simulink model "rcm112_app"  (R2024a)
settings: Solver=FixedStepDiscrete  StartTime=0.0  StopTime=10.0  FixedStep=0.005  RelTol=1e-3  EnableMultiTasking=on
PreLoadFcn:
  | try, model_open; catch, disp('Error occurred while executing model pre-load callback: model_open.m'); disp('Please assure that the MATLAB working directory is set to the model directory before opening.'); end
InitFcn:
  | try, model_open; catch, end
undefined symbols (not defined in the file or in its folder): dataName, enumName, enumValue, raptor_get_safe_string, raptor_xcp_function, RCM
libraries: Raptor_lib x57, simulink x14, simulink_extras x4
(part 1 of 2)
CloseFcn:
  | try, model_close; catch, end
settings Model: Raptor_Target=RCM-58NN-112-2202  Raptor_Calloc=NonVolatile (EEPROM)  RaptorUIDSize=4  RaptorBuildNum=1  Raptor_ecuaddr=11  Creator=mstewart  LastModifiedBy=mstewart
settings SolverCC: AlgebraicLoopSolver=TrustRegion
settings DataIOCC: LimitDataPoints=on  SaveFormat=Array  SignalLoggingSaveFormat=ModelDataLogs  ReturnWorkspaceOutputs=off
settings OptimizationCC: DefaultParameterBehavior=Inlined  ExpressionDepthLimit=2147483647  InitFltsAndDblsToZero=on  LifeSpan=1  EfficientTunableParamExpr=on
settings DebuggingCC: SolverPrmCheckMsg=warning  InheritedTsInSrcMsg=none  FcnCallInpInsideContextMsg=warning  UnconnectedInputMsg=warning  UnconnectedOutputMsg=warning  UnconnectedLineMsg=warning  StateNameClashWarn=warning  SFUnexpectedBacktrackingDiag=warning  SFNoUnconditionalDefaultTransitionDiag=warning  SFExecutionAtInitializationDiag=none  ArithmeticOperatorsInVariantConditions=warning
settings HardwareCC: ProdBitPerPointer=32  ProdBitPerSizeT=32  ProdBitPerPtrDiffT=32  ProdLargestAtomicInteger=Long  ProdLargestAtomicFloat=Double  ProdEndianess=BigEndian  ProdWordSize=32  ProdHWDeviceType=Freescale->MPC55xx  TargetIntDivRoundTo=Zero  TargetEndianess=BigEndian  ProdEqTarget=off
settings ModelReferenceCC: EnableRefExpFcnMdlSchedulingChecks=on  PropagateSignalLabelsOutOfModel=off
settings SFSimCC: SimUseLocalCustomCode=off  MATLABDynamicMemAlloc=off  CustomCodeUndefinedFunction=UseInterfaceOnly
settings RTWCC: Description=Raptor (tm)  SystemTargetFile=raptor.tlc  GenCodeOnly=on  MakeCommand=raptor_make_rtw  TemplateMakefile=raptor.tmf  RTWUseLocalCustomCode=off  GPUComputeCapability=3.5  DLArmComputeVersion=19.05
settings CodeAppCC: IgnoreCustomStorageClasses=off  MaxIdLength=100  CustomSymbolStrType=$N$R$M  StateflowObjectComments=on  InternalIdentifier=Classic
settings STFCustomTargetCC: TargetLangStandard=C89/C90 (ANSI)  CodeReplacementLibrary=No Double Hardware Support  GenerateSampleERTMain=on  ModelReferenceCompliant=off  CombineOutputUpdateFcns=on  ERTCustomFileBanners=on  SupportContinuousTime=off  SupportNonInlinedSFcns=off  RemoveResetFunc=on  MATLABClassNameForMDSCustomization=Simulink.SoftwareTarget.ERTCustomization  GRTInterface=off  UseToolchainInfoCompliant=off  SystemTargetFile=raptor.tlc
settings ERTTargetCC: CodeReplacementLibrary=No Double Hardware Support  MultiwordLength=2048  GenerateSampleERTMain=on  ModelReferenceCompliant=off  ParMdlRefBuildCompliant=off  CompOptLevelCompliant=off  ConcurrentExecutionCompliant=off  ModelStepFunctionPrototypeControlCompliant=off  CPPClassGenCompliant=off  UseToolchainInfoCompliant=off  ExtModeMexFile=noextcomm  InlinedParameterPlacement=NonHierarchical  ERTCustomFileTemplate=example_file_process.tlc  ConvertIfToSwitch=off  SuppressUnreachableDefaultCases=off
settings ConfigComp: CovMetricSettings=dw  CovSaveCumulativeToWorkspaceVar=on  CovSaveSingleToWorkspaceVar=on  CovExternalEMLEnable=off  CovSFcnEnable=off

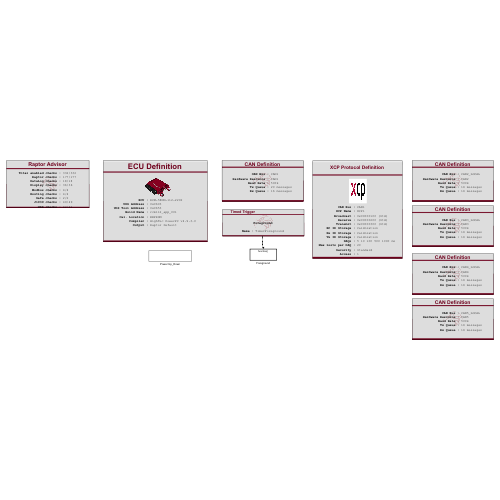
[thumbnail: Simulink's stored preview of the top-level diagram]
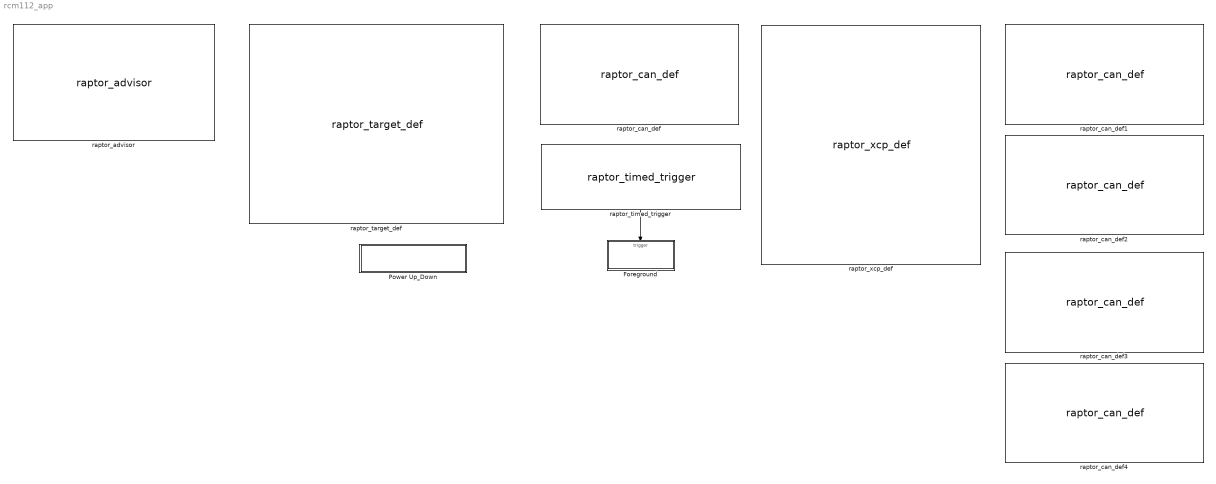
== system rcm112_app ==
  Foreground : Subsystem  TreatAsAtomicUnit=on
      settings: RTWSystemCode=Nonreusable function
  Power Up_Down : Subsystem  mask{group='Diagnostics | Power Up_Down'}
  raptor_advisor : Raptor_lib/Configuration/raptor_advisor  pop_setEnable=Enable All  ckb_Raptor=on  ckb_AppMonitor=on  tbl_AppMonitor={ 'on', 'App Monitor'; 'on', 'App Monitor Measurement'; 'on', 'App Monitor Stop'; 'on', 'Reboot'; 'on', 'Task Monitor'; 'on', 'Task Monitor Measurement' }  ckb_CAN=on  tbl_CAN={ 'on', 'CAN Baud Rate'; 'on', 'CAN Bus Off Recovery'; 'on', 'CAN Definition'; 'on', 'CAN Hardware Mailbox Config'; 'on', 'CAN Mailbox Properties'; 'on', 'CAN Partial Networking'; 'on', 'CAN Queue Info'; 'on', 'CAN Rx Message'; 'on', 'CAN Rx Raw'; 'on', 'CAN State'; 'on', 'CAN Trigger'; 'on', 'CAN Tx Message'; 'on', 'CAN Tx Raw'; 'on', 'CAN/FD Definition'; 'on', 'CAN/FD Rx Message'; 'on', 'CAN/FD Rx Raw'; 'on', 'CAN/FD Tx Message'; 'on', 'CAN/FD Tx Raw'; 'on', 'Custom Baud Rate'; 'on', 'DBC Pack'; 'on', 'DBC Unpack' }  ckb_Checksum=on  tbl_Checksum={ 'on', 'Calculate Checksum'; 'on', 'Read Checksum' }  ckb_Config=on  tbl_Config={ 'on', 'Configuration Read'; 'on', 'System Variable Access Level'; 'on', 'ECU Definition'; 'on', 'Set Target Address'; 'on', 'XCP Custom Security Seed/Key'; 'on', 'XCP Custom Security Trigger'; 'on', 'XCP Protocol Definition'; 'on', 'XCP Query'; 'on', 'XCP Set Address' }  ckb_DataStore=on  tbl_DataStore={ 'on', 'Adjustment'; 'on', 'Data Store'; 'on', 'Data Read'; 'on', 'Data Write'; 'on', 'Load NonVolatile Defaults'; 'on', 'Fixed NV Manager'; 'on', 'Measurement'; 'on', 'Memory Read'; 'on', 'NonVolatile Settings'; 'on', 'Override'; 'on', 'Fixed NonVolatile Status'; 'on', 'NonVolatile Status'; 'on', 'Store NonVolatile' }  ckb_Engine=on  tbl_Engine={ 'on', 'Angle Time'; 'on', 'CamShaft Sensor Info'; 'on', 'Encoder Def'; 'on', 'Injector Output'; 'on', 'Knock Results'; 'on', 'Knock Input'; 'on', 'Spark Output'; 'on', 'Wideband O2 Input' }  ckb_Ethernet=on  tbl_Ethernet={ 'on', 'Ethernet Adapter Get MAC Address'; 'on', 'Ethernet Definition'; 'on', 'Ethernet Interface Definition'; 'on', 'Ethernet Interface Get VLAN'; 'on', 'Ethernet Interface Set VLAN'; 'on', 'Ethernet Socket - TCP Server'; 'on', 'Ethernet Socket - UDP Server'; 'on', 'Ethernet Socket State'; 'on', 'Ethernet TCP Accept'; 'on', 'Ethernet TCP Close'; 'on', 'Ethernet TCP Connect'; 'on', 'Ethernet TCP Listen'; 'on', 'Ethernet TCP Receive'; 'on', 'Ethernet TCP Send'; 'on', 'Ethernet TCP Shutdown'; 'on', 'Ethernet UDP Multicast Join'; 'on', 'Ethernet UDP Multicast Leave'; 'on', 'Ethernet UDP Receive'; 'on', 'Ethernet UDP Send' }  ckb_OBD_Faults=on  tbl_OBD_Faults={ 'on', 'OBD Counter'; 'on', 'Increment OBD Counter'; 'on', 'Read OBD Counter'; 'on', 'Reset OBD Counter'; 'on', 'Drive Cycle Complete'; 'on', 'OBD Ratio'; 'on', 'Increment OBD Ratio'; 'on', 'Read OBD Ratio'; 'on', 'Reset OBD Ratio' }  ckb_Faults=on  tbl_Faults={ 'on', 'Fault Action'; 'on', 'Fault Action Iterator'; 'on', 'Fault Action Read'; 'on', 'Clear Fault'; 'on', 'Fault Data'; 'on', 'Fault Data Read'; 'on', 'Fault Data Write'; 'on', 'Fault'; 'on', 'Fault Handle'; 'on', 'Fault Iterator'; 'on', 'Fault Manager'; 'on', 'Fault Measurement'; 'on', 'Null Fault'; 'on', 'Fault Config'; 'on', 'Fault Reference'; 'on', 'Set Fault State'; 'on', 'Fault State Iterator'; 'on', 'Fault Status'; 'on', 'Fault Trigger'; 'on', 'Fault State Count' }  ckb_IO=on  tbl_IO={ 'on', 'Analog Input'; 'on', 'Analog Input Reference'; 'on', 'Analog Output'; 'on', 'Device Diagnostics'; 'on', 'Digital Input'; 'on', 'Digital Output'; 'on', 'Frequency Input'; 'on', 'H-Bridge Output'; 'on', 'IMU Calibrate'; 'on', 'IMU Reset'; 'on', 'IMU Status'; 'on', 'Inertial Measurement'; 'on', 'Input Capture Defn'; 'on', 'Input Capture Get'; 'on', 'Input Capture Trigger'; 'on', 'Input Status'; 'on', 'Internal Measurement'; 'on', 'Output Status'; 'on', 'PWM Output'; 'on', 'Quadrature Input'; 'on', 'Set Hardware Option'; 'on', 'Set Input Option'; 'on', 'Temperature Measurement' }  ckb_LIN=on  tbl_LIN={ 'on', 'LIN Master Definition'; 'on', 'LIN Get Schedule'; 'on', 'LIN Rx Message'; 'on', 'LIN Set Schedule'; 'on', 'LIN Slave Definition'; 'on', 'LIN State'; 'on', 'LIN Trigger'; 'on', 'LIN Tx Message' }  ckb_SENT=on  tbl_SENT={ 'on', 'SENT Definition'; 'on', 'SENT Receive State' }  ckb_Serial=on  tbl_Serial={ 'on', 'Serial Definition'; 'on', 'Serial Rx'; 'on', 'Serial Trigger'; 'on', 'Serial Tx' }  ckb_Strings=on  tbl_Strings={ 'on', 'String'; 'on', 'Arr 2 Str'; 'on', 'String Length'; 'on', 'Printf'; 'on', 'String Reference'; 'on', 'scanf'; 'on', 'Str 2 Arr' }  ckb_Tables=on  tbl_Tables={ 'on', 'Table Adapt'; 'on', 'Axis'; 'on', 'Axis Reference'; 'on', 'Table Interpolate 1D'; 'on', 'Table Interpolate 1D Reference'; 'on', 'Table Interpolate 2D'; 'on', 'Table Interpolate 2D Reference' }  ckb_Time=on  tbl_Time={ 'on', 'Datetime Conversion In'; 'on', 'Datetime Conversion Out'; 'on', 'Real Time Clock Read'; 'on', 'Real Time Clock Set' }  ckb_Triggers=on  tbl_Triggers={ 'on', 'App Trigger'; 'on', 'dT'; 'on', 'Distributed Action Defn'; 'on', 'Distributed Action Execute'; 'on', 'Distributed Action Trigger'; 'on', 'Shutdown'; 'on', 'Sleep'; 'on', 'Startup'; 'on', 'Time'; 'on', 'Timed Trigger'; 'on', 'Timed Trigger Config'; 'on', 'Define Trigger'; 'on', 'Trigger Execute'; 'on', 'Output Trigger Reference'; 'on', 'Trigger Select' }  ckb_DataLog=on  tbl_DataLog={ 'on', 'Data Log Erase'; 'on', 'Data Log Read'; 'on', 'Data Log Write'; 'on', 'File Close'; 'on', 'File EOF'; 'on', 'File Exists'; 'on', 'File Get Free Space'; 'on', 'File Open'; 'on', 'File Position'; 'on', 'File Read'; 'on', 'File Remove'; 'on', 'File Rename'; 'on', 'File Seek'; 'on', 'File Size'; 'on', 'File Sync'; 'on', 'USB Eject'; 'on', 'USB Status'; 'on', 'File Write' }  ckb_Display=on  ckb_Drawing=on  tbl_Drawing={ 'on', 'Clear Rect'; 'on', 'Clear Screen'; 'on', 'Draw Arc'; 'on', 'Draw Button'; 'on', 'Draw Circle'; 'on', 'Draw Image'; 'on', 'Draw Line'; 'on', 'Draw Polygon'; 'on', 'Draw Rectangle'; 'on', 'Draw Text'; 'on', 'Element'; 'on', 'Fill Circle'; 'on', 'Fill Ellipse'; 'on', 'Fill Polygon'; 'on', 'Fill Rect'; 'on', 'Image Ref' }  ckb_Menu=on  tbl_Menu={ 'on', 'Menu Screen Definition'; 'on', 'Menu Sel Item'; 'on', 'Menu Text'; 'on', 'Menu Title' }  ckb_Prefab=on  tbl_Prefab={ 'on', 'Gauge: Create'; 'on', 'Gauge: Update' }  ckb_ScreenFuncs=on  tbl_ScreenFuncs={ 'on', 'Hide Buttonbar'; 'on', 'Button Bar Properties'; 'on', 'Setup Button'; 'on', 'Goto Screen'; 'on', 'Recalibrate Screen'; 'on', 'Screen Definition'; 'on', 'Screen Reference'; 'on', 'Screen Select'; 'on', 'Splash Screen' }  ckb_Touchscreen=on  tbl_Touchscreen={ 'on', 'Button Status'; 'on', 'Display Touchscreen'; 'on', 'Button Def'; 'on', 'Hot Area Actions'; 'on', 'Update Swipe Action' }  ckb_Modbus=on  tbl_Modbus={ 'on', 'Modbus Master'; 'on', 'Modbus Slave'; 'on', 'Modbus Slave Error'; 'on', 'Modbus Slave Response' }  ckb_Routing=on  tbl_Routing={ 'on', 'J1939 Message Router'; 'on', 'Message Hardware Filter'; 'on', 'Message Network'; 'on', 'Message Router' }  ckb_Safe=on  tbl_Safe={ 'on', 'Raptor Stack Check'; 'on', 'Raptor Time Check' }  ckb_J1939=on  ckb_DMA=on  tbl_DMA={ 'on', 'DM14/15/16 Definition: DM14 Rx'; 'on', 'DM14/15/16 Definition: DM15 Rx'; 'on', 'DM14/15/16 Definition: DM15 Tx'; 'on', 'DM14/15/16 Definition: DMA Manager'; 'on', 'DMA Address Space Definition'; 'on', 'DMA Address Space Return'; 'on', 'DMA Address Space Trigger'; 'on', 'DMA Key'; 'on', 'DMA Key Trigger' }  ckb_DM_Msgs=on  tbl_DM_Msgs={ 'on', 'DM4 Transmit'; 'on', 'DM5 Transmit'; 'on', 'DM8 Transmit'; 'on', 'DM19 Transmit'; 'on', 'DM20 Transmit'; 'on', 'DM21 Transmit'; 'on', 'DM22 Rx Trigger'; 'on', 'DM24 Transmit'; 'on', 'DM25 Transmit'; 'on', 'DM26 Transmit'; 'on', 'DM29 Transmit'; 'on', 'DM30 Transmit'; 'on', 'DM33 Transmit'; 'on', 'DM34 Transmit'; 'on', 'DTC Transmit' }  ckb_EFF=on  tbl_EFF={ 'on', 'Clear Expanded FF'; 'on', 'Write Expanded FF'; 'on', 'Expanded FF Status' }  ckb_PGN_Tx=on  tbl_PGN_Tx={ 'on', 'CBI Transmit'; 'on', 'CI Transmit'; 'on', 'EC1 Transmit'; 'on', 'ECUID Transmit'; 'on', 'GTFI Transmit'; 'on', 'LTFI Transmit'; 'on', 'RC Transmit'; 'on', 'SOFT Transmit'; 'on', 'TTI2 Transmit'; 'on', 'VI Transmit' }  ckb_SPN=on  tbl_SPN={ 'on', 'SPN Read'; 'on', 'SPN Write' }  ckb_J1939_TP=on  tbl_J1939_TP={ 'on', 'J1939 DTC Rx Handler'; 'on', 'Source Addr'; 'on', 'PGN Enable'; 'on', 'PGN Request Slot'; 'on', 'PGN Enable'; 'on', 'PGN Trigger'; 'on', 'Tx ACK/NACK'; 'on', 'J1939 Protocol'; 'on', 'J1939 Transport Protocol Receive'; 'on', 'PGN Rx Trigger' }  ckb_UDS=on  ckb_ISO14229=on  tbl_ISO14229={ 'on', 'ISO14229 Custom Service 0x31'; 'on', 'ISO14229 Service 0x10 - Session Control'; 'on', 'ISO14229 Service 0x11 - ECU Reset'; 'on', 'ISO14229 Service 0x14 - Clear Diagnostic Information'; 'on', 'ISO14229 Service 0x19 - Read DTC Information'; 'on', 'ISO14229 Service 0x19 - Extended Data Definition'; 'on', 'ISO14229 Service 0x19 - Snapshot Record Definition'; 'on', 'ISO14229 Service 0x19 - Snapshot Record Clear'; 'on', 'ISO14229 Service 0x19 - Snapshot Record Clear All'; 'on', 'ISO14229 Service 0x19 - Snapshot Record Get'; 'on', 'ISO14229 Service 0x19 - Snapshot Record Set'; 'on', 'ISO14229 Service 0x22 - Read Data by Identifier'; 'on', 'ISO14229 Service 0x27 - Security Access'; 'on', 'ISO14229 Service 0x28 - Communication Control'; 'on', 'ISO14229 Service 0x2E - Write Data by Identifier'; 'on', 'ISO14229 Service 0x2F - Input Output by Identifier'; 'on', 'ISO14229 Service 0x2F - Input Output by Identifier Reset State'; 'on', 'ISO14229 Service 0x31 - Routine Control by Identifier'; 'on', 'ISO14229 Service 0x85 - DTC Control Setting' }  ckb_ISO15031=on  tbl_ISO15031={ 'on', 'ISO15031 Custom Service'; 'on', 'ISO15031 Service 0x01'; 'on', 'ISO15031 Service 0x03 - Emission-related diagnostic trouble codes'; 'on', 'ISO15031 Service 0x04 - Clear Diagnostic Information'; 'on', 'ISO15031 Service 0x07 - Emission-related pending diagnostic trouble codes'; 'on', 'ISO15031 Service 0x09 - Calibration Identification'; 'on', 'ISO15031 Service 0x09 - Calibration Verification Numbers'; 'on', 'ISO15031 Service 0x09 - ECU Name'; 'on', 'ISO15031 Service 0x09 - Request Vehicle Information'; 'on', 'ISO15031 Service 0x09 - Vehicle Identification Number'; 'on', 'ISO15031 Service 0x0A - Emission-related diagnostic trouble codes with permanent status' }  ckb_ISO15765=on  tbl_ISO15765={ 'on', 'ISO15765 Protocol Receive Queue Info'; 'on', 'ISO15765 Protocol Transmit Queue Info'; 'on', 'ISO15765 Protocol Transmit Raw' }  ckb_UDS_Basics=on  tbl_UDS_Basics={ 'on', 'UDS Client Functional Address Request'; 'on', 'UDS Client Functional Address Request Send'; 'on', 'UDS Protocol Client Request Raw'; 'on', 'UDS Protocol Receive Raw'; 'on', 'UDS Protocol Transmit Raw'; 'on', 'UDS Server Service Process Raw' }  ckb_UDS_Other=on  tbl_UDS_Other={ 'on', 'ISO13400 DoIP Entity'; 'on', 'UDS Protocol'; 'on', 'UDS Set Buffer Storage' }
      settings: SourceProductName=Raptor
  raptor_can_def : Raptor_lib/CAN/raptor_can_def  canBus='CAN1'  resourceValues=CAN5|CAN1|CAN2|CAN3|CAN4|(None)  resource=CAN1  baudRateValues=33k|50k|100k|125k|200k|250k|333k|500k|667k|800k|1000k|500k_80%SP|500k_81%SP  baudRate=500k  enable_baud_rate_config=0  sim_func_name='ConfigureCANBaudRate'  createButton=0  txQueueSize=20  rxQueueSize=16  useCustomBR=0  customBR='CustomBaudRate'  updateButton=0
      settings: SourceProductName=Raptor
  raptor_can_def1 : Raptor_lib/CAN/raptor_can_def  canBus='CAN2_LOCAL'  resourceValues=CAN5|CAN1|CAN2|CAN3|CAN4|(None)  resource=CAN2  baudRateValues=33k|50k|100k|125k|200k|250k|333k|500k|667k|800k|1000k  baudRate=500k  enable_baud_rate_config=0  sim_func_name='ConfigureCANBaudRate'  createButton=[]  txQueueSize=16  rxQueueSize=16  useCustomBR=0  customBR='CustomBaudRate'  updateButton=[]
      settings: SourceProductName=Raptor
  raptor_can_def2 : Raptor_lib/CAN/raptor_can_def  canBus='CAN3_LOCAL'  resourceValues=CAN5|CAN1|CAN2|CAN3|CAN4|(None)  resource=CAN3  baudRateValues=33k|50k|100k|125k|200k|250k|333k|500k|667k|800k|1000k  baudRate=500k  enable_baud_rate_config=0  sim_func_name='ConfigureCANBaudRate'  createButton=[]  txQueueSize=16  rxQueueSize=16  useCustomBR=0  customBR='CustomBaudRate'  updateButton=[]
      settings: SourceProductName=Raptor
  raptor_can_def3 : Raptor_lib/CAN/raptor_can_def  canBus='CAN4_LOCAL'  resourceValues=CAN5|CAN1|CAN2|CAN3|CAN4|(None)  resource=CAN4  baudRateValues=33k|50k|100k|125k|200k|250k|333k|500k|667k|800k|1000k  baudRate=500k  enable_baud_rate_config=0  sim_func_name='ConfigureCANBaudRate'  createButton=[]  txQueueSize=16  rxQueueSize=16  useCustomBR=0  customBR='CustomBaudRate'  updateButton=[]
      settings: SourceProductName=Raptor
  raptor_can_def4 : Raptor_lib/CAN/raptor_can_def  canBus='CAN5_LOCAL'  resourceValues=CAN5|CAN1|CAN2|CAN3|CAN4|(None)  resource=CAN5  baudRateValues=33k|50k|100k|125k|200k|250k|333k|500k|667k|800k|1000k  baudRate=500k  enable_baud_rate_config=0  sim_func_name='ConfigureCANBaudRate'  createButton=[]  txQueueSize=16  rxQueueSize=16  useCustomBR=0  customBR='CustomBaudRate'  updateButton=[]
      settings: SourceProductName=Raptor
  raptor_target_def : Raptor_lib/Configuration/raptor_target_def  targetValues=BCM-5606B-060-2201|BCM-5646-48-1404|CSM-S32K148-030-1903|DISP-VC128-1901|DISP-VC320L-1402|DISP-VC320-1204|DISP-VC800-1402|DISP-VC500-1904|DISP-VC700-2003|DISP-VC300R-2004|GCM-5634M-070-1459|GCM-5634M-070-1559|GCM-5634M-070-1562|ECM-1793-196-1503|GCM-1793-196-1503|GCM-5605B-048-1906|GCM-5605B-048-2104|GCM-5607B-80-1901|GCM-5607B-80-1903|GCM-5607B-80-2001|RCM-5743R-080-2005|RCM-5743R-080-2106|RCM-5743R-080-2203|UAS-5743R-047-2102|UAS-5743R-047-2107|GCM-5746R-048-1902|RCM-58NN-112-2007|RCM-58NN-112-2103|RCM-58NN-112-2202|HCM-5604-36-1303|HCM-5604-36-1702  target=RCM-58NN-112-2202  simpack=0  simulator=0  heap=4*1024  stack=2*1024  fgndStack=3*1024  bgndStack=2*1024  idleStack=1024  intStack=1536  sdStack=1024  appStack=1024  ecuaddr=11  uds_server_addr_ext=0  uds_server_addr=hex2dec('603')  uds_client_addr=hex2dec('653')  callocValues=Constant (FLASH)|NonVolatile (EEPROM)  calloc=NonVolatile (EEPROM)  compilerValues=HighTec PowerPC v4.9.3.0|SPC5Studio-6.0.0-Green  compiler=HighTec PowerPC v4.9.3.0  setFileName=0  exeName=[raptor_get_safe_string(bdroot) '_']  addBuildNum=1  minVerChars=3  extraOutput=0  buildLocationValues=Raptor Default|Model Directory|User Defined  buildLocation=Raptor Default  exeLocation=''  exeFileButton=0  a2lLocation=''  a2lFileButton=0  rpgLocation=''  rpgFileButton=0
      settings: SourceProductName=Raptor
  raptor_timed_trigger : Raptor_lib/Triggers/raptor_timed_trigger  triggerValues=Task_Core0_1ms|Task_Core0_5ms|Task_Core0_10ms|Task_Core0_20ms|Task_Core0_50ms|Task_Core0_100ms|Task_Core0_250ms|Task_Core0_500ms|Second|Minute|Foreground|Background  trigger=Foreground  inherited=0  alwaysEnabled=1  triggerPriority=0  triggerName=Foreground
      settings: SourceProductName=Raptor
  raptor_xcp_def : Raptor_lib/Configuration/raptor_xcp_def  XCPname='XCP1'  canBus='CAN1'  bcID=hex2dec('100')  bcID_TypeValues=Standard|Extended  bcID_Type=Standard  rxID=hex2dec('200')  rxID_TypeValues=Standard|Extended  rxID_Type=Standard  txID=hex2dec('300')  txID_TypeValues=Standard|Extended  txID_Type=Standard  daqRates=[5 10 100 500 1000]  numODTs=20  genCANAPE=0  genVISION=0  securityValues=Standard|None|Custom User Defined|LoopEnergy  security=Standard  dllName=raptor_XCPSecurity.dll  accessValues=4|3|2|1  access=1  bcStorageValues=Constant (FLASH)|NonVolatile (EEPROM)|FixedNonVolatile (EEPROM)|Volatile (RAM)|Calibration  bcStorage=Calibration  txStorageValues=Constant (FLASH)|NonVolatile (EEPROM)|FixedNonVolatile (EEPROM)|Volatile (RAM)|Calibration  txStorage=Calibration  rxStorageValues=Constant (FLASH)|NonVolatile (EEPROM)|FixedNonVolatile (EEPROM)|Volatile (RAM)|Calibration  rxStorage=Calibration
      settings: SourceProductName=Raptor
  wires:
  raptor_timed_trigger/1 -> Foreground/Trigger

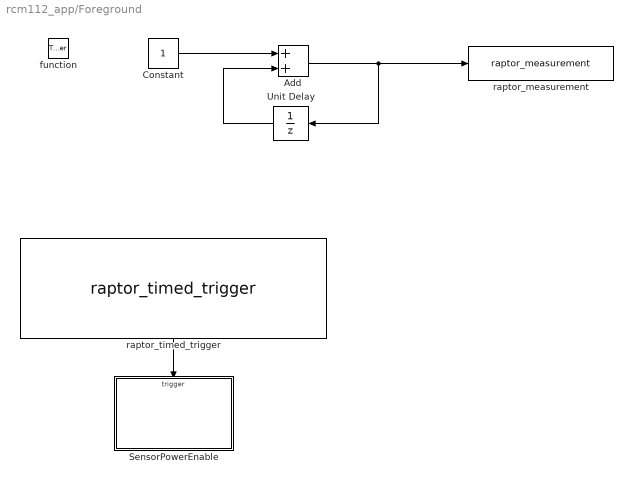
== system rcm112_app/Foreground ==
  function : TriggerPort  TriggerType=function-call  VariantControl=Variant
  Add : Sum
  Constant : Constant
  SensorPowerEnable : Subsystem
  Unit Delay : UnitDelay  SampleTime=-1  HasFrameUpgradeWarning=on
  raptor_measurement : Raptor_lib/Data Storage/raptor_measurement  paramName='Counter'  nameSource=Parameter  calDispType=Number  calEnum={'False', 'True'}  calGain=1.0  calOffset=0.0  calMax=inf  calMin=-inf  calFormat='-1'  calUnit=''  calHelp=''  calAccess=4  calFunction=raptor_xcp_function(gcb)  calVisible=on
      settings: SourceProductName=Raptor
  raptor_timed_trigger : Raptor_lib/Triggers/raptor_timed_trigger  triggerValues=Task_Core0_1ms|Task_Core0_Fgnd|Task_Core0_20ms|Task_Core0_50ms|Task_Core0_100ms|Task_Core0_250ms|Task_Core0_500ms|Second|Minute|Foreground|Foregroundx2|Foregroundx5|Foregroundx10|Foregroundx20|Background|Backgroundx2|Backgroundx5|Backgroundx10|Backgroundx20  trigger=Task_Core0_Fgnd  inherited=1  alwaysEnabled=1  triggerPriority=0  triggerName=FGND_10MS_SensPower
      settings: SourceProductName=Raptor
  wires:
  Constant/1 -> Add/1
  Add/1 -> raptor_measurement/1, Unit Delay/1
  Unit Delay/1 -> Add/2
  raptor_timed_trigger/1 -> SensorPowerEnable/Trigger

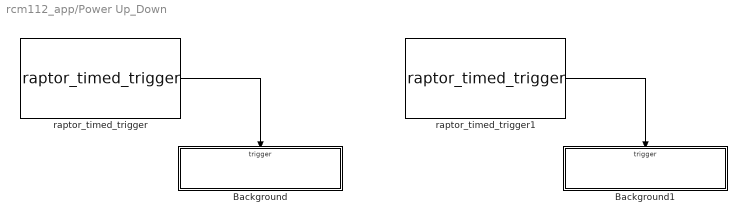
== system rcm112_app/Power Up_Down ==
  Background : Subsystem  mask{group='System | Power Up_Down', samptime=.05}
      mask prompts: samptime "Sample Time"
      mask Display: disp(['Sample Time:\n' num2str(samptime)])
  Background1 : Subsystem
  raptor_timed_trigger : Raptor_lib/Triggers/raptor_timed_trigger  triggerValues=Task_Core0_1ms|Task_Core0_5ms|Task_Core0_10ms|Task_Core0_20ms|Task_Core0_50ms|Task_Core0_100ms|Task_Core0_250ms|Task_Core0_500ms|Second|Minute|Foreground|Background  trigger=Background  inherited=0  alwaysEnabled=1  triggerPriority=50  triggerName=Background_50MS
      settings: SourceProductName=Raptor
  raptor_timed_trigger1 : Raptor_lib/Triggers/raptor_timed_trigger  triggerValues=Task_Core0_1ms|Task_Core0_5ms|Task_Core0_10ms|Task_Core0_20ms|Task_Core0_50ms|Task_Core0_100ms|Task_Core0_250ms|Task_Core0_500ms|Second|Minute|Foreground|Background  trigger=Background  inherited=0  alwaysEnabled=1  triggerPriority=51  triggerName=Background_50MS_SBN1H
      settings: SourceProductName=Raptor
  wires:
  raptor_timed_trigger/1 -> Background/Trigger
  raptor_timed_trigger1/1 -> Background1/Trigger

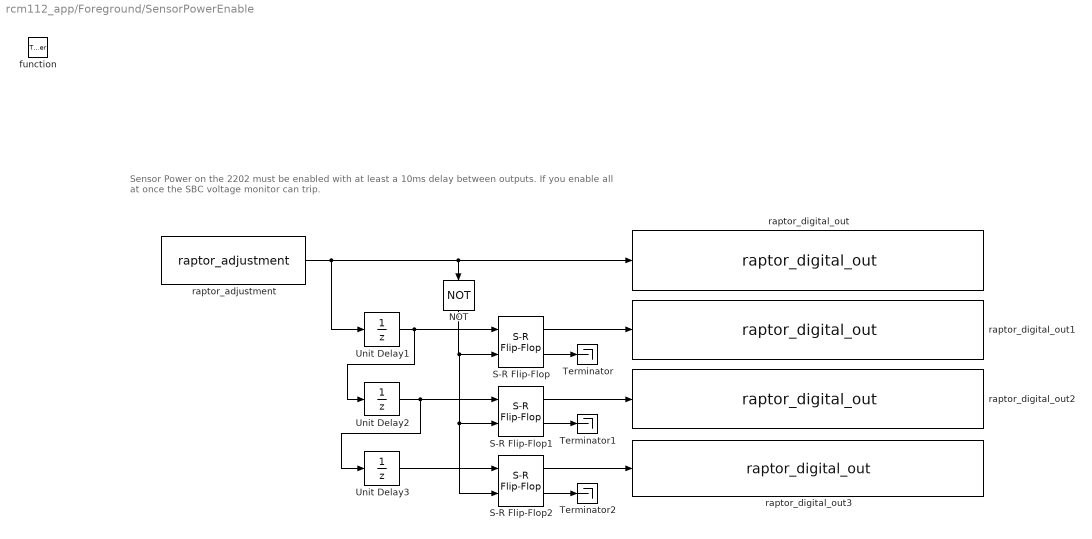
== system rcm112_app/Foreground/SensorPowerEnable ==
  note: Sensor Power on the 2202 must be enabled with at least a 10ms delay between outputs. If you enable all at once the SBC voltage monitor can trip.
  function : TriggerPort  TriggerType=function-call  VariantControl=Variant
  NOT : Logic  Operator=NOT
  S-R Flip-Flop : simulink_extras/Flip Flops/S-R Flip-Flop  initial_condition=0
  S-R Flip-Flop1 : simulink_extras/Flip Flops/S-R Flip-Flop  initial_condition=0
  S-R Flip-Flop2 : simulink_extras/Flip Flops/S-R Flip-Flop  initial_condition=0
  Terminator : Terminator
  Terminator1 : Terminator
  Terminator2 : Terminator
  Unit Delay1 : UnitDelay  SampleTime=-1  HasFrameUpgradeWarning=on
  Unit Delay2 : UnitDelay  SampleTime=-1  HasFrameUpgradeWarning=on
  Unit Delay3 : UnitDelay  SampleTime=-1  HasFrameUpgradeWarning=on
  raptor_adjustment : Raptor_lib/Data Storage/raptor_adjustment  paramName='SensorPowerEnable'  nameSource=Parameter  initValue=false  dataType=boolean  storage=Calibration  calDispType=Enumeration  calEnum={'False', 'True'}  calGain=1.0  calOffset=0.0  calMax=inf  calMin=-inf  calFormat='-1'  calUnit=''  calHelp=''  calAccess=1  calFunction='Enables'  calDispHeaders=off  calColHeaders={'Col1' 'Col2' 'Col3'}  calRowHeaders={'Row1' 'Row2' 'Row3'}
      settings: SourceProductName=Raptor
  raptor_digital_out : Raptor_lib/Input & Output/raptor_digital_out  resourceValues=SENSOR_POWER_A_EN|SENSOR_POWER_B_EN|SENSOR_POWER_C_EN|SENSOR_POWER_D_EN|LSO1|MPRD_EN|POWER_HOLD|(None)  resource=SENSOR_POWER_A_EN  driverTypeValues=Enable  driverType=Enable
      settings: SourceProductName=Raptor
  raptor_digital_out1 : Raptor_lib/Input & Output/raptor_digital_out  resourceValues=SENSOR_POWER_A_EN|SENSOR_POWER_B_EN|SENSOR_POWER_C_EN|SENSOR_POWER_D_EN|LSO1|MPRD_EN|POWER_HOLD|(None)  resource=SENSOR_POWER_B_EN  driverTypeValues=Enable  driverType=Enable
      settings: SourceProductName=Raptor
  raptor_digital_out2 : Raptor_lib/Input & Output/raptor_digital_out  resourceValues=SENSOR_POWER_A_EN|SENSOR_POWER_B_EN|SENSOR_POWER_C_EN|SENSOR_POWER_D_EN|LSO1|MPRD_EN|POWER_HOLD|(None)  resource=SENSOR_POWER_C_EN  driverTypeValues=Enable  driverType=Enable
      settings: SourceProductName=Raptor
  raptor_digital_out3 : Raptor_lib/Input & Output/raptor_digital_out  resourceValues=SENSOR_POWER_A_EN|SENSOR_POWER_B_EN|SENSOR_POWER_C_EN|SENSOR_POWER_D_EN|LSO1|MPRD_EN|POWER_HOLD|(None)  resource=SENSOR_POWER_D_EN  driverTypeValues=Enable  driverType=Enable
      settings: SourceProductName=Raptor
  wires:
  S-R Flip-Flop/1 -> raptor_digital_out1/1
  Unit Delay1/1 -> S-R Flip-Flop/1, Unit Delay2/1
  raptor_adjustment/1 -> NOT/1, raptor_digital_out/1, Unit Delay1/1
  NOT/1 -> S-R Flip-Flop2/2, S-R Flip-Flop1/2, S-R Flip-Flop/2
  S-R Flip-Flop/2 -> Terminator/1
  S-R Flip-Flop1/2 -> Terminator1/1
  S-R Flip-Flop2/1 -> raptor_digital_out3/1
  S-R Flip-Flop1/1 -> raptor_digital_out2/1
  Unit Delay2/1 -> S-R Flip-Flop1/1, Unit Delay3/1
  Unit Delay3/1 -> S-R Flip-Flop2/1
  S-R Flip-Flop2/2 -> Terminator2/1

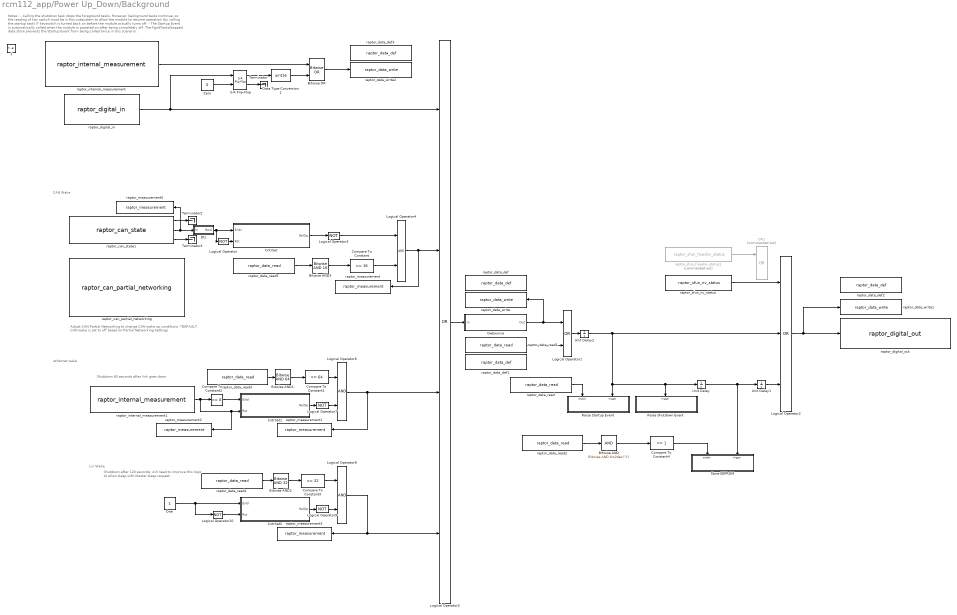
== system rcm112_app/Power Up_Down/Background ==
  note: Shutdown 60 seconds after link goes down
  note: ethernet wake
  note: Notes :
      | - Calling the shutdown task stops the foreground tasks. However, background tasks continue, so the reading of key switch must be in this subsystem to allow the module
      | to resume operation (by calling the startup task) if keyswitch is turned back on before the module actually turns off.
      | - The Startup Event is automatically called when the module is powered on after being completely off. The FgndTasksStopped data store prevents the Startup Event from being called twice in this scenario.
  note: CAN Wake
  note: Lin Wake
  note: Shutdown after 120 seconds; will need to improve this logic to allow sleep with Master sleep request.
  note: Adjust CAN Partial Networking to change CAN wake up conditions.
      | *DEFAULT CAN wake is set to off based on Partial Networking Settings.
  f : TriggerPort  TriggerType=function-call  VariantControl=Variant  ZeroCross=off
  Bitwise AND : simulink/Logic and Bit Operations/Bitwise Operator  logicop=AND  UseBitMask=on  BitMask=bin2dec('1')  BitMaskRealWorld=Stored Integer
  Bitwise AND1 : simulink/Logic and Bit Operations/Bitwise Operator  logicop=AND  UseBitMask=on  BitMask=64  BitMaskRealWorld=Stored Integer
  Bitwise AND2 : simulink/Logic and Bit Operations/Bitwise Operator  logicop=AND  UseBitMask=on  BitMask=32  BitMaskRealWorld=Stored Integer
  Bitwise AND3 : simulink/Logic and Bit Operations/Bitwise Operator  logicop=AND  UseBitMask=on  BitMask=16  BitMaskRealWorld=Stored Integer
  Bitwise OR : simulink/Logic and Bit Operations/Bitwise Operator  logicop=OR  UseBitMask=off  NumInputPorts=2  BitMask=bin2dec('11011001')  BitMaskRealWorld=Stored Integer
  CntrSat : Subsystem  mask(CntrSat){init=0, timeout=60, inc=1, typ=uint32, relop=>=, th_nam='Wake_CAN5_SleepDelayTime', th_help='make sure this is long enough that we dont trigger a ton of EEPROM writes between messages', th_units='sec', th_gain=samptime, th_group=group}
      mask prompts: init "Initial Value (after a reset)"; inc "Increment"; typ "Data Type"; relop "Relational Operator"; th_nam "Thresh. Name"; th_help "Thresh. Help Text"; th_units "Thresh. Units"; th_gain "Thresh. Gain"; th_group "Thresh. Group"
      mask init:
      | cb = gcb;
      | 
      | % --- Parameter Setting
      | set_param([cb '/Relational Operator'], 'Operator', relop);
      | set_param([cb '/raptor_adjustment'], 'dataType', typ);
      | set_param([cb '/Constant'], 'OutDataTypeStr', typ);
      | set_param([cb '/Constant1'], 'OutDataTypeStr', typ);
      | 
      | % --- Precision
      | try
      |     th_gain_eval = raptor_get_param_eval(th_gain);
      |     inc_eval = raptor_get_param_eval(inc);
      |     prec = SamptimePrec(th_gain_eval * inc_eval);
      | catch
      |     prec = '';
      | end
      mask TypeOptions typ: double | single | int8 | uint8 | int16 | uint16 | int32 | uint32 | boolean
      mask TypeOptions relop: == | >= | >
      mask Display: disp(['Counter\n' typ '\n' relop ' ' th_nam]);
  CntrSat1 : Subsystem  mask(CntrSat){init=0, timeout=60, inc=1, typ=uint32, relop=>=, th_nam='Wake_ETH_SleepDelayTime', th_help='make sure this is long enough that we dont trigger a ton of EEPROM writes between messages', th_units='sec', th_gain=samptime, th_group=group}
      mask prompts: init "Initial Value (after a reset)"; inc "Increment"; typ "Data Type"; relop "Relational Operator"; th_nam "Thresh. Name"; th_help "Thresh. Help Text"; th_units "Thresh. Units"; th_gain "Thresh. Gain"; th_group "Thresh. Group"
      mask init: same as rcm112_app/Power Up_Down/Background/CntrSat
      mask TypeOptions typ: double | single | int8 | uint8 | int16 | uint16 | int32 | uint32 | boolean
      mask TypeOptions relop: == | >= | >
      mask Display: disp(['Counter\n' typ '\n' relop ' ' th_nam]);
  CntrSat2 : Subsystem  mask(CntrSat){init=0, timeout=60, inc=1, typ=uint32, relop=>=, th_nam='Wake_LIN2_SleepDelayTime', th_help='make sure this is long enough that we dont trigger a ton of EEPROM writes between messages', th_units='sec', th_gain=samptime, th_group=group}
      mask prompts: init "Initial Value (after a reset)"; inc "Increment"; typ "Data Type"; relop "Relational Operator"; th_nam "Thresh. Name"; th_help "Thresh. Help Text"; th_units "Thresh. Units"; th_gain "Thresh. Gain"; th_group "Thresh. Group"
      mask init: same as rcm112_app/Power Up_Down/Background/CntrSat
      mask TypeOptions typ: double | single | int8 | uint8 | int16 | uint16 | int32 | uint32 | boolean
      mask TypeOptions relop: == | >= | >
      mask Display: disp(['Counter\n' typ '\n' relop ' ' th_nam]);
  Compare To Constant : simulink/Logic and Bit Operations/Compare To Constant  relop===  const=16  OutDataTypeStr=boolean
  Compare To Constant1 : simulink/Logic and Bit Operations/Compare To Constant  relop===  const=64  OutDataTypeStr=boolean
  Compare To Constant2 : simulink/Logic and Bit Operations/Compare To Constant  relop===  const=0  OutDataTypeStr=boolean
  Compare To Constant3 : simulink/Logic and Bit Operations/Compare To Constant  relop===  const=32  OutDataTypeStr=boolean
  Compare To Constant4 : simulink/Logic and Bit Operations/Compare To Constant  relop===  const=1  OutDataTypeStr=boolean
  Data Type Conversion1 : DataTypeConversion  OutDataTypeStr=uint16  SaturateOnIntegerOverflow=off  RndMeth=Floor
  Debounce : Subsystem
  Dtc : Subsystem  mask(Dtc){init=0, relop===}
      mask prompts: init "Initial Condition (of input):"; relop "Relational Operator"
      mask init:
      | cb = gcb;
      | 
      | % --- Parameter Setting
      | set_param([cb '/Relational Operator'], 'Operator', relop);
      mask TypeOptions relop: == | ~= | < | <= | >= | >
      mask Display: disp(['U ' relop ' U/z']);
  Logical Operator{,3,7,9..10} (5 alike) : Logic  Operator=NOT  AllPortsSameDT=off  OutDataTypeStr=boolean
  Logical Operator1 : Logic  Operator=OR  OutDataTypeStr=boolean
  Logical Operator2 : Logic  Operator=OR  Inputs=3  OutDataTypeStr=boolean
  Logical Operator4 : Logic  AllPortsSameDT=off  OutDataTypeStr=boolean
  Logical Operator5 : Logic  Operator=OR  Inputs=4  OutDataTypeStr=boolean
  Logical Operator6 : Logic  AllPortsSameDT=off  OutDataTypeStr=boolean
  Logical Operator8 : Logic  AllPortsSameDT=off  OutDataTypeStr=boolean
  OR1 : Logic  Commented=on  Operator=OR
  One : Constant  OutDataTypeStr=Inherit: Inherit via back propagation
  Raise Shutdown Event : Subsystem  TreatAsAtomicUnit=on
  Raise Startup Event : Subsystem  TreatAsAtomicUnit=on
  S-R Flip-Flop : simulink_extras/Flip Flops/S-R Flip-Flop  initial_condition=0
  Store EEPROM : Subsystem  TreatAsAtomicUnit=on
  Terminator : Terminator
  Terminator2 : Terminator
  Terminator3 : Terminator
  Unit Delay : UnitDelay  SampleTime=-1  HasFrameUpgradeWarning=on
  Unit Delay1 : UnitDelay  SampleTime=-1  HasFrameUpgradeWarning=on
  Unit Delay2 : UnitDelay  InitialCondition=1  SampleTime=-1  HasFrameUpgradeWarning=on
  Zero : Constant  Value=0  OutDataTypeStr=boolean
  raptor_can_partial_networking : Raptor_lib/CAN/raptor_can_partial_networking  resourceValues=CAN5  resource=CAN5  CANid=hex2dec('7FF')  ID_TypeValues=Standard|Extended  ID_Type=Standard  CANmask=hex2dec('7FF')  data=[0x00 0x00 0x00 0x00 0x00 0x00 0x00 0x00]  dataLength=8
      settings: SourceProductName=Raptor
  raptor_can_state1 : Raptor_lib/CAN/raptor_can_state  resourceValues=CAN5|CAN1|CAN2|CAN3|CAN4|(None)  resource=CAN5
      settings: SourceProductName=Raptor
  raptor_data_def : Raptor_lib/Data Storage/raptor_data_def  dataName='KeySw_Bgnd'  initValue=0  dataType=boolean  storage=Volatile (RAM)  calVisible=on  calType=Measurement  calDispType=Number  calEnum={'False', 'True'}  calGain=1.0  calOffset=0  calMin=-Inf  calMax=Inf  calFormat='-1'  calUnit='Bool'  calHelp='Key switch reading from background task'  calAccess=1  calFunction=group  calDispHeaders=off  calColHeaders={'Col1' 'Col2' 'Col3'}  calRowHeaders={'Row1' 'Row2' 'Row3'}
      settings: SourceProductName=Raptor
  raptor_data_def1 : Raptor_lib/Data Storage/raptor_data_def  dataName='KeepModuleOn'  initValue=0  dataType=boolean  storage=Volatile (RAM)  calVisible=on  calType=Measurement  calDispType=Number  calEnum={'False', 'True'}  calGain=1.0  calOffset=0  calMin=-Inf  calMax=Inf  calFormat='-1'  calUnit='Bool'  calHelp='Boolean indicating module to be kept on'  calAccess=1  calFunction=group  calDispHeaders=off  calColHeaders={'Col1' 'Col2' 'Col3'}  calRowHeaders={'Row1' 'Row2' 'Row3'}
      settings: SourceProductName=Raptor
  raptor_data_def2 : Raptor_lib/Data Storage/raptor_data_def  dataName='MPRD_EN'  initValue=0  dataType=boolean  storage=Volatile (RAM)  calVisible=on  calType=Measurement  calDispType=Number  calEnum={'False', 'True'}  calGain=1.0  calOffset=0  calMin=-Inf  calMax=Inf  calFormat='-1'  calUnit='Bool'  calHelp='Enable signal for Main Power Relay Driver.'  calAccess=1  calFunction=group  calDispHeaders=off  calColHeaders={'Col1' 'Col2' 'Col3'}  calRowHeaders={'Row1' 'Row2' 'Row3'}
      settings: SourceProductName=Raptor
  raptor_data_def3 : Raptor_lib/Data Storage/raptor_data_def  dataName='Wake_Source'  initValue=0  dataType=uint16  storage=Volatile (RAM)  calVisible=on  calType=Measurement  calDispType=Number  calEnum={'False', 'True'}  calGain=1.0  calOffset=0  calMin=-Inf  calMax=Inf  calFormat='-1'  calUnit='BITFeild'  calHelp='Source of the Current Wake.'  calAccess=1  calFunction=group  calDispHeaders=off  calColHeaders={'Col1' 'Col2' 'Col3'}  calRowHeaders={'Row1' 'Row2' 'Row3'}
      settings: SourceProductName=Raptor
  raptor_data_read : Raptor_lib/Data Storage/raptor_data_read  dataName='FgndTasksStopped'  dataShape=Scalar  idxSource=Input  idxRow=1  idxCol=1
      settings: SourceProductName=Raptor
  raptor_data_read1 : Raptor_lib/Data Storage/raptor_data_read  dataName='KeepModuleOn'  dataShape=Scalar  idxSource=Input  idxRow=1  idxCol=1
      settings: SourceProductName=Raptor
  raptor_data_read{2..5} (4 alike) : Raptor_lib/Data Storage/raptor_data_read  dataName='Wake_Source'  dataShape=Scalar  idxSource=Input  idxRow=1  idxCol=1
      settings: SourceProductName=Raptor
  raptor_data_write : Raptor_lib/Data Storage/raptor_data_write  dataName='KeySw_Bgnd'  dataShape=Scalar  idxSource=Input Port  idxRow=1  idxCol=1
      settings: SourceProductName=Raptor
  raptor_data_write1 : Raptor_lib/Data Storage/raptor_data_write  dataName='MPRD_EN'  dataShape=Scalar  idxSource=Input Port  idxRow=1  idxCol=1
      settings: SourceProductName=Raptor
  raptor_data_write2 : Raptor_lib/Data Storage/raptor_data_write  dataName='Wake_Source'  dataShape=Scalar  idxSource=Input Port  idxRow=1  idxCol=1
      settings: SourceProductName=Raptor
  raptor_digital_in : Raptor_lib/Input & Output/raptor_digital_in  resourceValues=(None)|WAKE_INPUT1|INPUT33|INPUT34|INPUT35|INPUT36|INPUT37|INPUT38|INPUT39|INPUT40  resource=WAKE_INPUT1  pullUDValues=2.9k PD  pullUD=(None)  upperThres=1.980  lowerThres=1.320
      settings: SourceProductName=Raptor
  raptor_digital_out : Raptor_lib/Input & Output/raptor_digital_out  resourceValues=OUTPUT9|OUTPUT21|OUTPUT22|OUTPUT23|OUTPUT24|(None)|OUTPUT1|OUTPUT2|OUTPUT3|OUTPUT4|OUTPUT5|OUTPUT6|OUTPUT7|OUTPUT8|OUTPUT10|OUTPUT11|OUTPUT25|OUTPUT26|OUTPUT27|OUTPUT28|OUTPUT29|OUTPUT30|OUTPUT31|OUTPUT32|OUTPUT33|OUTPUT34|OUTPUT35|OUTPUT36|OUTPUT37|OUTPUT38|OUTPUT39|OUTPUT40|OUTPUT41|OUTPUT42|OUTPUT43|OUTPUT44|OUTPUT45|OUTPUT46|OUTPUT47|OUTPUT48|POWER_HOLD  resource=POWER_HOLD  driverTypeValues=(None)  driverType=Enable
      settings: SourceProductName=Raptor
  raptor_internal_measurement : Raptor_lib/Input & Output/raptor_internal_measurement  Priority=0  resourceValues=MPRD_FDBK|DRVP|HB1P_HSO_CURRENT|HB1P_LSO_CURRENT|HB1M_HSO_CURRENT|HB1M_LSO_CURRENT|HB2P_HSO_CURRENT|HB2P_LSO_CURRENT|HB2M_HSO_CURRENT|HB2M_LSO_CURRENT|WAKE_SOURCE|SENSOR_POWER_A|SENSOR_POWER_B|SENSOR_POWER_C|SENSOR_POWER_D|VBATT|HSO1_CURRENT|HSO2_CURRENT|HSO3_CURRENT|HSO4_CURRENT|LSO1_CURRENT|LSO2_CURRENT|LSO3_CURRENT|LSO4_CURRENT|LSO5_CURRENT|LSO6_CURRENT|LSO7_CURRENT|LSO8_CURRENT|EthLinkStatus|CPU0IdleUtilization  resource=WAKE_SOURCE  out_eng=0  soft_filter=1  out_bool=0
      settings: SourceProductName=Raptor
  raptor_internal_measurement1 : Raptor_lib/Input & Output/raptor_internal_measurement  resourceValues=MPRD_FDBK|DRVP|HB1P_HSO_CURRENT|HB1P_LSO_CURRENT|HB1M_HSO_CURRENT|HB1M_LSO_CURRENT|HB2P_HSO_CURRENT|HB2P_LSO_CURRENT|HB2M_HSO_CURRENT|HB2M_LSO_CURRENT|WAKE_SOURCE|SENSOR_POWER_A|SENSOR_POWER_B|SENSOR_POWER_C|SENSOR_POWER_D|VBATT|HSO1_CURRENT|HSO2_CURRENT|HSO3_CURRENT|HSO4_CURRENT|LSO1_CURRENT|LSO2_CURRENT|LSO3_CURRENT|LSO4_CURRENT|LSO5_CURRENT|LSO6_CURRENT|LSO7_CURRENT|LSO8_CURRENT|EthLinkStatus|CPU0IdleUtilization  resource=EthLinkStatus  out_eng=1  soft_filter=1  out_bool=1
      settings: SourceProductName=Raptor
  raptor_measurement : Raptor_lib/Data Storage/raptor_measurement  paramName='CANWakeIndicator'  nameSource=Parameter  calDispType=Number  calEnum={'False', 'True'}  calGain=1.0  calOffset=0.0  calMax=inf  calMin=-inf  calFormat='-1'  calUnit=''  calHelp=''  calAccess=1  calFunction=group  calVisible=on
      settings: SourceProductName=Raptor
  raptor_measurement1 : Raptor_lib/Data Storage/raptor_measurement  paramName='EthWakeIndicator'  nameSource=Parameter  calDispType=Number  calEnum={'False', 'True'}  calGain=1.0  calOffset=0.0  calMax=inf  calMin=-inf  calFormat='-1'  calUnit=''  calHelp=''  calAccess=1  calFunction=group  calVisible=on
      settings: SourceProductName=Raptor
  raptor_measurement2 : Raptor_lib/Data Storage/raptor_measurement  paramName='EthLinkStatus'  nameSource=Parameter  calDispType=Number  calEnum={'False', 'True'}  calGain=1.0  calOffset=0.0  calMax=inf  calMin=-inf  calFormat='-1'  calUnit=''  calHelp=''  calAccess=1  calFunction=group  calVisible=on
      settings: SourceProductName=Raptor
  raptor_measurement3 : Raptor_lib/Data Storage/raptor_measurement  paramName='LINWakeIndicator'  nameSource=Parameter  calDispType=Number  calEnum={'False', 'True'}  calGain=1.0  calOffset=0.0  calMax=inf  calMin=-inf  calFormat='-1'  calUnit=''  calHelp=''  calAccess=1  calFunction=group  calVisible=on
      settings: SourceProductName=Raptor
  raptor_measurement5 : Raptor_lib/Data Storage/raptor_measurement  paramName='Wake_CAN5_RxCount'  nameSource=Parameter  calDispType=Number  calEnum={'False', 'True'}  calGain=1.0  calOffset=0.0  calMax=inf  calMin=-inf  calFormat='-1'  calUnit=''  calHelp=''  calAccess=4  calFunction=group  calVisible=on
      settings: SourceProductName=Raptor
  raptor_sfun_fixednv_status1 : Raptor_lib/Data Storage/raptor_sfun_fixednv_status  Commented=on  showStatus=Store In Progess
      settings: SourceProductName=Raptor
  raptor_sfun_nv_status : Raptor_lib/Data Storage/raptor_sfun_nv_status  showStatus=Store In Progess
      settings: SourceProductName=Raptor
  wires:
  CntrSat/1(RelOp) -> Logical Operator3/1
  raptor_data_read1/1 -> Logical Operator1/2
  Unit Delay1/1 -> Logical Operator2/3
  Logical Operator2/1 -> raptor_data_write1/1, raptor_digital_out/1
  Logical Operator4/1 -> raptor_measurement/1, Logical Operator5/2
  raptor_data_read/1 -> Raise Startup Event/Enable
  Logical Operator1/1 -> Unit Delay2/1
  raptor_can_state1/3 -> Terminator3/1
  Logical Operator3/1 -> Logical Operator4/1
  Logical Operator/1 -> CntrSat/2(Rst)
  raptor_can_state1/1 -> Terminator2/1
  raptor_can_state1/2 -> raptor_measurement5/1, Dtc/1(In)
  Dtc/1(Bool) -> CntrSat/1(Enbl), Logical Operator/1
  Unit Delay2/1 -> Raise Startup Event/Trigger, Raise Shutdown Event/Trigger, Unit Delay/1, Logical Operator2/2
  Compare To Constant/1 -> Logical Operator4/2
  Compare To Constant1/1 -> Logical Operator6/1
  CntrSat1/1(RelOp) -> Logical Operator7/1
  Logical Operator7/1 -> Logical Operator6/2
  Logical Operator6/1 -> raptor_measurement1/1, Logical Operator5/3
  Logical Operator5/1 -> Debounce/1(In)
  Debounce/1(Out) -> raptor_data_write/1, Logical Operator1/1
  Unit Delay/1 -> Store EEPROM/Trigger, Unit Delay1/1
  Compare To Constant2/1 -> CntrSat1/1(Enbl)
  raptor_internal_measurement1/1 -> raptor_measurement2/1, CntrSat1/2(Rst), Compare To Constant2/1
  Logical Operator8/1 -> Logical Operator5/4, raptor_measurement3/1
  Logical Operator9/1 -> Logical Operator8/2
  CntrSat2/1(RelOp) -> Logical Operator9/1
  Compare To Constant3/1 -> Logical Operator8/1
  Logical Operator10/1 -> CntrSat2/2(Rst)
  One/1 -> CntrSat2/1(Enbl), Logical Operator10/1
  raptor_data_read2/1 -> Bitwise AND/1
  Compare To Constant4/1 -> Store EEPROM/Enable
  raptor_data_read3/1 -> Bitwise AND1/1
  raptor_data_read4/1 -> Bitwise AND2/1
  raptor_internal_measurement/1 -> Bitwise OR/1
  raptor_data_read5/1 -> Bitwise AND3/1
  Bitwise AND/1 -> Compare To Constant4/1
  Bitwise AND1/1 -> Compare To Constant1/1
  Bitwise AND2/1 -> Compare To Constant3/1
  Bitwise AND3/1 -> Compare To Constant/1
  Bitwise OR/1 -> raptor_data_write2/1
  S-R Flip-Flop/1 -> Data Type Conversion1/1
  Zero/1 -> S-R Flip-Flop/2
  S-R Flip-Flop/2 -> Terminator/1
  raptor_digital_in/1 -> S-R Flip-Flop/1, Logical Operator5/1
  Data Type Conversion1/1 -> Bitwise OR/2
  raptor_sfun_nv_status/1 -> Logical Operator2/1
  raptor_sfun_fixednv_status1/1 -> OR1/1

== system rcm112_app/Power Up_Down/Background1 ==
  note: Notes :
      | - Calling the shutdown task stops the foreground tasks. However, background tasks continue, so the reading of key switch must be in this subsystem to allow the module
      | to resume operation (by calling the startup task) if keyswitch is turned back on before the module actually turns off.
      | - The Startup Event is automatically called when the module is powered on after being completely off. The FgndTasksStopped data store prevents the Startup Event from being called twice in this scenario.
  f : TriggerPort  TriggerType=function-call  VariantControl=Variant  ZeroCross=off
  raptor_data_read1 : Raptor_lib/Data Storage/raptor_data_read  dataName='MPRD_EN'  dataShape=Scalar  idxSource=Input  idxRow=1  idxCol=1
      settings: SourceProductName=Raptor
  raptor_digital_out1 : Raptor_lib/Input & Output/raptor_digital_out  resourceValues=LSO1|MPRD_EN|POWER_HOLD|SENSOR_POWER_EN|(None)  resource=MPRD_EN  driverTypeValues=Enable  driverType=Enable
      settings: SourceProductName=Raptor
  wires:
  raptor_data_read1/1 -> raptor_digital_out1/1

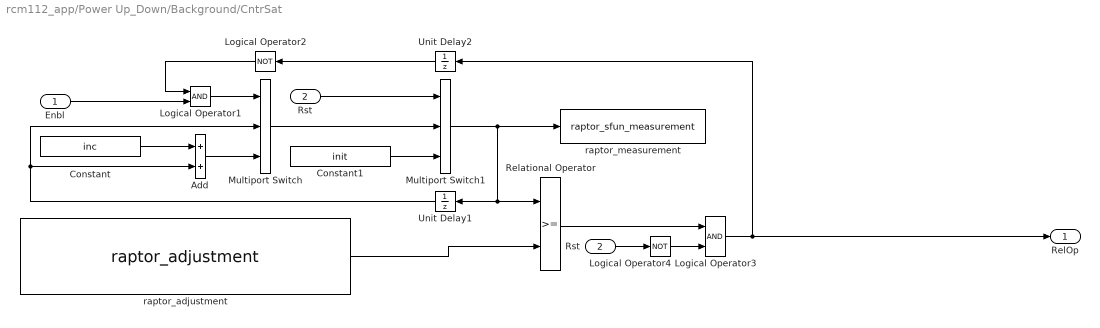
== system rcm112_app/Power Up_Down/Background/CntrSat ==
  Enbl : Inport
  Rst : Inport  Port=2
  Add : Sum  InputSameDT=on  OutDataTypeStr=Inherit: Same as first input
  Constant : Constant  Value=inc  OutDataTypeStr=uint32
  Constant1 : Constant  Value=init  OutDataTypeStr=uint32
  Logical Operator1 : Logic  OutDataTypeStr=boolean
  Logical Operator2 : Logic  Operator=NOT  Inputs=1  OutDataTypeStr=boolean
  Logical Operator3 : Logic  OutDataTypeStr=boolean
  Logical Operator4 : Logic  Operator=NOT  Inputs=1  OutDataTypeStr=boolean
  Multiport Switch : MultiPortSwitch  DataPortOrder=Zero-based contiguous  Inputs=2  zeroidx=on  SaturateOnIntegerOverflow=off
  Multiport Switch1 : MultiPortSwitch  DataPortOrder=Zero-based contiguous  Inputs=2  zeroidx=on  SaturateOnIntegerOverflow=off
  Relational Operator : RelationalOperator  OutDataTypeStr=boolean  InputSameDT=off
  "Rst " : InportShadow  Port=2
  Unit Delay1 : UnitDelay  InitialCondition=init  SampleTime=-1  HasFrameUpgradeWarning=on
  Unit Delay2 : UnitDelay  InitialCondition=boolean(0)  SampleTime=-1  HasFrameUpgradeWarning=on
  raptor_adjustment : Raptor_lib/Data Storage/raptor_adjustment  paramName=th_nam  nameSource=Parameter  initValue=timeout / th_gain  dataType=uint32  storage=Calibration  calDispType=Number  calEnum={'Disabled', 'Enabled'}  calGain=th_gain  calOffset=0  calMax=inf  calMin=-inf  calFormat='0.3'  calUnit=th_units  calHelp=th_help  calAccess=4  calFunction=th_group  calDispHeaders=off  calColHeaders={'Col1' 'Col2' 'Col3'}  calRowHeaders={'Row1' 'Row2' 'Row3'}
      settings: SourceProductName=Raptor
  raptor_measurement : S-Function  FunctionName=raptor_sfun_measurement  Parameters=char({dataName,''}), uint8(calDispType), char(enumName), int32(enumValue), double(calGain), double(calOffset), double(calMax), double(calMin), char(calUnit), char(calHelp), char(calFormat), char(calFunction), char(calAccess)  SFunctionDeploymentMode=off  EnableBusSupport=off  mask(Measurement){paramName=[th_nam(1:end-3) 'Tmr'], nameSource=Parameter, calDispType=Number, calEnum={'False', 'True'}, calGain=th_gain, calOffset=0.0, calMax=inf, calMin=-inf, calFormat='0.3', calUnit=th_units, calHelp=['time that gets compared to ' th_nam], calAccess=4, calFunction=th_group, calVisible=on}
      mask prompts: paramName "Name"; nameSource "Name Source"; calDispType "Display as"; calEnum "Enumeration Definition"; calGain "Gain"; calOffset "Offset"; calMax "Max"; calMin "Min"; calFormat "Display Decimal Places"; calUnit "Unit Text"; calHelp "Help Text"; calAccess "Access Level"; calFunction "Function"; calVisible "Visible in Cal"
      mask help: This block is used to display a value in the calibration tool.
      mask init:
      | raptor_sfun_measurement_maskInit;
      settings: MoveFcn=raptor_icon_redraw(gcb);
      mask Help: eval('raptor_help(''raptor_measurement'');')
      mask TypeOptions nameSource: Parameter | Input Wire
      mask Callback nameSource: raptor_sfun_measurement_dlgCb(gcb, 'nameSource');
      mask TypeOptions calDispType: Number | Enumeration | String
      mask Callback calDispType: raptor_sfun_measurement_dlgCb(gcb, 'calDispType');
      mask TypeOptions calAccess: 4 | 3 | 2 | 1
      mask Display: raptor_sfun_measurement_icon;
  RelOp : Outport  VectorParamsAs1DForOutWhenUnconnected=off
  wires:
  Unit Delay2/1 -> Logical Operator2/1
  Rst/1 -> Multiport Switch1/1
  Logical Operator3/1 -> Unit Delay2/1, RelOp/1
  raptor_adjustment/1 -> Relational Operator/2
  Enbl/1 -> Logical Operator1/2
  Logical Operator1/1 -> Multiport Switch/1
  Add/1 -> Multiport Switch/3
  Unit Delay1/1 -> Add/2, Multiport Switch/2
  Constant/1 -> Add/1
  Multiport Switch/1 -> Multiport Switch1/2
  Constant1/1 -> Multiport Switch1/3
  Logical Operator2/1 -> Logical Operator1/1
  Multiport Switch1/1 -> raptor_measurement/1, Unit Delay1/1, Relational Operator/1
  Relational Operator/1 -> Logical Operator3/1
  Logical Operator4/1 -> Logical Operator3/2
  "Rst "/1 -> Logical Operator4/1
